simulink model "SparkEV"  (R2022b)
settings: configuration reference "VehicleVariableDae" (kept outside this file)
StartFcn:
  | %tic
StopFcn:
  | %toc
undefined symbols (not defined in the file): CtrlTcuInitGear, CtrlVcuCltch1InitCmd, Disabled, DriverPreviewDist, EnvAbsPrs, EnvAirTemp, EnvGrvty, EnvNomFrictionScaling, EnvNominalGrade, EnvWindVelX, EnvWindVelY, EnvWindVelZ, PlntVehDstCGFrntAxl, PlntVehDstCGRearAxl, PlntVehInitLatPos, PlntVehInitLongPos, PlntVehInitPitchAng, PlntVehInitRollAng, PlntVehInitVertPos, PlntVehInitYawAng, PlntVehMass, PlntVehTrckWdth, PlntVehYawMomentInertia, ScnCRMaxLatAccel, ScnCRRadius, ScnDLCGateLongPos, ScnDLCLatRef, ScnDLCLatRefOffset, ScnDLCLongRefBpt, ScnDLCLongRefStartPos, ScnDLCVehicleWidth, ScnFHCounterDwellTime, ScnFHInitialDwellTime, ScnFHReturnTime, ScnFHRollRateZeroCross, ScnFHSteerAmp, ScnFHSteerSpeed, ScnISHandwheelRate, ScnISMaxHandwheelAng, ScnISMaxLatAccel, ScnISSteerHoldTime, ScnLongVelRef, ScnSDDwellTime, ScnSDSteerAmp, ScnSDSteerFreq, ScnSimTime, ScnSSFinalFreq, ScnSSSteerAmp, ScnSSSweepTime, ScnStartTime, US06
libraries: simulink x13, vehdynlibscenariocommon x7, vehdynlibviscommon x3, autolibshared x2, sim3dgroundtruthsensorlib x2, vehdynlibdriver x1, sharedtransform x1, sim3dlib x1, sim3dautolib x1
(part 3 of 4)

== system SparkEV/Driver Commands/Driver Commands/Open Loop ==
  VehFdbk : Inport
  SteerCmd : Inport  Port=2
  AccelCmd : Inport  Port=3
  BrakeCmd : Inport  Port=4
  GearCmd : Inport  Port=5
  Bus Creator1 : BusCreator  Inputs=5
  Constant : Constant  Value=false
  Signal Specification : SignalSpecification  Unit=1
  Signal Specification1 : SignalSpecification  Unit=1
  Signal Specification2 : SignalSpecification  Unit=1
  Terminator : Terminator
  Unit Conversion : UnitConversion
  Wheel Angle Limit * Steer Ratio : Gain  Gain=40*pi/180*18
  Driver : Outport  VectorParamsAs1DForOutWhenUnconnected=off
  wires:
  Signal Specification2/1 -> Bus Creator1/4  "GearCmd"
  BrakeCmd/1 -> Signal Specification1/1
  Wheel Angle Limit * Steer Ratio/1 -> Bus Creator1/1  "SteerCmd"
  Bus Creator1/1 -> Driver/1
  Unit Conversion/1 -> Wheel Angle Limit * Steer Ratio/1
  AccelCmd/1 -> Signal Specification/1
  VehFdbk/1 -> Terminator/1
  SteerCmd/1 -> Unit Conversion/1
  Signal Specification/1 -> Bus Creator1/2  "AccelCmd"
  GearCmd/1 -> Signal Specification2/1
  Signal Specification1/1 -> Bus Creator1/3  "DecelCmd"
  Constant/1 -> Bus Creator1/5  "IgnSwtch"

== system SparkEV/Driver Commands/Driver Commands/Predictive Driver ==
  VehRef : Inport
  VehFdbk : Inport  Port=2
  Env : Inport  Port=3
  Bus Creator1 : BusCreator  Inputs=5
  Bus Selector : BusSelector  OutputSignals=Body.InertFrm.Cg.Disp.Y,Body.BdyFrm.Cg.Vel.ydot,Body.InertFrm.Cg.Ang.psi,Body.BdyFrm.Cg.AngVel.r
  Bus Selector1 : BusSelector  OutputSignals=LngRef,LtrlRef,EnblSteerCmd,SteerOvrCmd,SteerHld,SteerZero,EnblAccelOvr,AccelOvrCmd,AccelHld,AccelZero,EnblDecelCmd,DecelOvrCmd,DecelHld,DecelZero
  Constant : Constant  Value=false
  Hill Hold : Subsystem
  Linear Predictive Driver : vehdynlibdriver/Predictive Driver  extAccelOvr=on  extDecelOvr=on  extAccelHld=on  extDecelHld=on  extAccelZero=on  extDecelZero=on  extSteerOvr=on  extSteerHld=on  extSteerZero=on  cntrlType=Predictive  cntrlTypeLat=Predictive  shftType=Reverse, Neutral, Drive  coordMode=SAE J670 (Z-down)  refType=Reference pose  velUnits=m/s  angUnits=rad  gearOut=on  steerOut=on  Kp=3  Ki=1  Kff=1  Kg=0  VehVelVec=[0 100]  KffVec=[.1 .1]  KpVec=[10 10]  KiVec=[5 5]  KgVec=[0 0]  vnom=5  Kaw=1  tauerr=.075  tau=DriverTimeConst  L=DriverPreviewDist  Kpt=DriverTractiveForce  aR=DriverRollRes  bR=DriverDrivelineRes  cR=DriverAeroRes  g=EnvGrvty  vecPose=off  dynamMode=off  PositionGainF=2.5  PositionGainR=2.5  YawRateGain=.2  DelayGain=.2  enableDrift=off  BetaRef=10  KpBeta=1  KpDrift=1  KdDrift=1  KpPsi=1  KOmega=.1  tOmega=.1  a=PlntVehDstCGFrntAxl  b=PlntVehDstCGRearAxl  m=PlntVehMass  Cy_f=DriverFrontCornerStiff  Cy_r=DriverRearCornerStiff  I=PlntVehYawMomentInertia  Ksteer=PlntSteerRatio  theta=DriverWheelRange  Idl=1  Re=PlntWhlLdRadius  lambda_mu=1  GearInit=DriverInitialGear  tShift=DriverShiftTime  pdlVec=[0.1 0.4 0.5 0.9]  upShftTbl=[-1 12.9375 26.4375 39.9375 51.18749999999999 62.4375 72.84375 83.25;-1 16.3125 29.8125 43.3125 54.5624 65.8125 76.78125 87.75;-1 19.6875 33.1875 46.68749999999999 57.9375 69.1875 80.71875 92.25;-1 33 52.5 77.25 100.5 138.75 161.875 185]  dwnShftTbl=[-1 12.9375 26.4375 39.9375 51.18749999999999 62.4375 72.84375 83.25;-1 16.3125 29.8125 43.3125 54.5624 65.8125 76.78125 87.75;-1 19.6875 33.1875 46.68749999999999 57.9375 69.1875 80.71875 92.25;-1 33 52.5 77.25 100.5 138.75 161.875 185]  tClutch=.5  tRev=.5  tPark=120  UpGearVec="[0  1  2  3  4  5  6  7]"  DownGearVec="[1  2  3  4  5  6  7  8]"  aMode=2
  Terminator : Terminator
  Unit Conversion : UnitConversion
  Driver : Outport  VectorParamsAs1DForOutWhenUnconnected=off
  wires:
  Linear Predictive Driver/3 -> Bus Creator1/2  "AccelCmd"
  Bus Selector/2 -> Linear Predictive Driver/18  "<ydot>"
  Bus Selector/1 -> Linear Predictive Driver/17  "<Y>"
  Bus Selector1/10 -> Linear Predictive Driver/10  "<AccelZero>"
  Bus Creator1/1 -> Driver/1
  Linear Predictive Driver/1 -> Terminator/1
  Bus Selector/3 -> Linear Predictive Driver/19  "<psi>"
  VehFdbk/1 -> Hill Hold/7(VehFdbk), Bus Selector/1
  Bus Selector1/2 -> Linear Predictive Driver/2  "<LtrlRef>"
  Bus Selector/4 -> Linear Predictive Driver/20  "<r>"
  VehRef/1 -> Bus Selector1/1
  Bus Selector1/1 -> Unit Conversion/1  "<LngRef>"
  Linear Predictive Driver/2 -> Bus Creator1/1  "SteerCmd"
  Linear Predictive Driver/4 -> Bus Creator1/3  "DecelCmd"
  Linear Predictive Driver/5 -> Bus Creator1/4  "GearCmd"
  Constant/1 -> Bus Creator1/5  "IgnSwtch"
  Bus Selector1/3 -> Linear Predictive Driver/3  "<EnblSteerCmd>"
  Bus Selector1/4 -> Linear Predictive Driver/4  "<SteerOvrCmd>"
  Bus Selector1/5 -> Linear Predictive Driver/5  "<SteerHld>"
  Bus Selector1/6 -> Linear Predictive Driver/6  "<SteerZero>"
  Bus Selector1/7 -> Linear Predictive Driver/7  "<EnblAccelOvr>"
  Bus Selector1/8 -> Linear Predictive Driver/8  "<AccelOvrCmd>"
  Bus Selector1/9 -> Linear Predictive Driver/9  "<AccelHld>"
  Bus Selector1/11 -> Hill Hold/2(<EnblDecelCmd>)  "<EnblDecelCmd>"
  Bus Selector1/12 -> Hill Hold/3(<DecelOvrCmd>)  "<DecelOvrCmd>"
  Bus Selector1/13 -> Hill Hold/4(<DecelHld>)  "<DecelHld>"
  Bus Selector1/14 -> Hill Hold/5(<DecelZero>)  "<DecelZero>"
  Env/1 -> Hill Hold/6(Env)
  Hill Hold/5(Grade) -> Linear Predictive Driver/15
  Hill Hold/6(VelFdbk) -> Linear Predictive Driver/16
  Hill Hold/4(DecelZero) -> Linear Predictive Driver/14
  Hill Hold/3(DecelHld) -> Linear Predictive Driver/13
  Hill Hold/2(DecelOvrCmd) -> Linear Predictive Driver/12
  Hill Hold/1(EnblDecelOvr) -> Linear Predictive Driver/11
  Unit Conversion/1 -> Linear Predictive Driver/1, Hill Hold/1(LngRef)

== system SparkEV/Environment/Ground Feedback/3D Engine ==
  Friction : Inport
  WheelFdbk : Inport  Port=2
  3D Engine Source : Subsystem  Variant=on  VariantControl=Choice  mask(Terrain Source){terrType=Single point}
      mask prompts: terrType "Terrain feedback type:"
      mask help:
      | This variant subsystem provides the option for:
      | - a single point of contact for each wheel with minimal post-processing ideal for smooth surfaces and maximum run-time performance.
      | - multiple points of contact per wheel which may be used when interested in non-smooth terrain at a higher computational cost and requires Vehicle Dynamics Blockset.
      mask TypeOptions terrType: Single point | Multiple points
  Bus Creator2 : BusCreator  Inputs=4
  Bus Creator3 : BusCreator  Inputs=3
  Demux1 : Demux
  Signal Specification1 : SignalSpecification  Unit=1
  Ground : Outport  VectorParamsAs1DForOutWhenUnconnected=off
  wires:
  Signal Specification1/1 -> Demux1/1
  Demux1/1 -> Bus Creator2/1  "mu_FL"
  Demux1/3 -> Bus Creator2/3  "mu_RL"
  Demux1/4 -> Bus Creator2/4  "mu_RR"
  Demux1/2 -> Bus Creator2/2  "mu_FR"
  Bus Creator2/1 -> Bus Creator3/3  "mu"
  Bus Creator3/1 -> Ground/1
  Friction/1 -> Signal Specification1/1
  WheelFdbk/1 -> 3D Engine Source/1(WheelFdbk)
  3D Engine Source/1(z) -> Bus Creator3/1  "z"
  3D Engine Source/2(DCM) -> Bus Creator3/2  "DCM"

== system SparkEV/Environment/Ground Feedback/Constant ==
  Friction : Inport
  Bus Creator : BusCreator  Inputs=4
  Bus Creator2 : BusCreator  Inputs=4
  Bus Creator3 : BusCreator  Inputs=3
  Constant1 : Constant  Value=zeros(4,1)
  Constant2 : Constant  Value=repmat(eye(3),1,1,4)  SampleTime=-1
  Demux : Demux
  Demux1 : Demux
  Signal Specification : SignalSpecification  Unit=m
  Signal Specification1 : SignalSpecification  Unit=1
  Ground : Outport  VectorParamsAs1DForOutWhenUnconnected=off
  wires:
  Constant1/1 -> Signal Specification/1
  Signal Specification/1 -> Demux/1
  Demux/4 -> Bus Creator/4  "G_RR_z"
  Demux/1 -> Bus Creator/1  "G_FL_z"
  Demux/3 -> Bus Creator/3  "G_RL_z"
  Demux/2 -> Bus Creator/2  "G_FR_z"
  Bus Creator/1 -> Bus Creator3/1  "z"
  Demux1/3 -> Bus Creator2/3  "mu_RL"
  Demux1/4 -> Bus Creator2/4  "mu_RR"
  Demux1/1 -> Bus Creator2/1  "mu_FL"
  Demux1/2 -> Bus Creator2/2  "mu_FR"
  Bus Creator2/1 -> Bus Creator3/3  "mu"
  Friction/1 -> Signal Specification1/1
  Signal Specification1/1 -> Demux1/1
  Bus Creator3/1 -> Ground/1
  Constant2/1 -> Bus Creator3/2  "DCM"

== system SparkEV/Environment/Varying Friction/Constant Friction ==
  Friction Scaling : Constant  Value=ones(4,1).*EnvNomFrictionScaling  SampleTime=0
  FricCoeffLambda : Outport
  wires:
  Friction Scaling/1 -> FricCoeffLambda/1

== system SparkEV/Environment/Varying Friction/Varying Friction ==
  In1 : Inport
  In2 : Inport  Port=2
  Cg : Inport  Port=3
  Bus Selector : BusSelector  OutputSignals=FrntAxl.Lft.Disp.X,FrntAxl.Rght.Disp.X,RearAxl.Lft.Disp.X,RearAxl.Rght.Disp.X
  Bus Selector1 : BusSelector  OutputSignals=FrntAxl.Lft.Disp.Y,FrntAxl.Rght.Disp.Y,RearAxl.Lft.Disp.Y,RearAxl.Rght.Disp.Y
  Road Track Friction : Subsystem  mask(Road Track Friction){surface_popup=Split friction coefficient scaling factor, lambda_g=EnvNomFrictionScaling, lambda_r=.6, r_x0=175, r_y0=-100, r_xw=1000, r_yw=500, aMode=2}
      mask prompts: surface_popup "Type of surface:"; lambda_g "Scaling factor for the friction coefficient of ground, lambda_g :"; lambda_r "Scaling factor for the friction coefficient of rectangular surface, lambda_r :"; r_x0 "X coordinate of lower left corner of rectangular surface, r_x0 [m]:"; r_y0 "Y coordinate of lower left corner of rectangular surface, r_y0 [m]:"; r_xw "Rectangular surface width in X direction, r_xw [m]:"; r_yw "Rectangular surface width in Y direction, r_yw [m]:"
      mask init:
      | % Scaling factor for the friction coefficient around the rectangular region
      | mutable = [lambda_g, lambda_g, lambda_g, lambda_g;
      |            lambda_g, lambda_r, lambda_r, lambda_g; 
      |            lambda_g, lambda_r, lambda_r, lambda_g; 
      |            lambda_g, lambda_g, lambda_g, lambda_g ];
      |        
      | 
      | % The step is distance between breakpoint near the boundary of high and
      | % low friction coefficient
      | 
      | step = 0.01 ; 
      | 
      | % In the mask initialization, xbr and ybr breakpoints are with respect to
      | % Body fixed coordinate system. At time t=0, xbr and ybr breakpoints
      | % updates to Earth (Inertial) Fixed coordinate system. The breakpoints for
      | % the lookup table are added via inputs.
      | 
      | xbr = [(r_x0 - step) , (r_x0 + step), (r_x0 + r_xw - step) , (r_x0 + r_xw + step) ];
      | ybr = [(r_y0 - step) , (r_y0 + step), (r_y0 + r_yw - step) , (r_y0 + r_yw + step) ];
      | 
      | 
      | % To check if the created track is split mu or constant mu
      | 
      | surface_popup = get_param(gcb, 'surface_popup');
      | 
      | if strcmp(surface_popup, 'Split friction coefficient scaling factor')
      |     SplitLambdaTrck = 1;
      | elseif strcmp(surface_popup, 'Constant friction coefficient scaling factor')
      |     SplitLambdaTrck = 0;
      | end
      mask Help: eval('vdynblkshelp(''vdynblkstrack'')');
      mask TypeOptions surface_popup: Constant friction coefficient scaling factor | Split friction coefficient scaling factor
      mask Callback surface_popup:
      | surface_popup = get_param(gcb, 'surface_popup');
      | m = Simulink.Mask.get(gcb);
      | 
      | lambda_g = m.getParameter('lambda_g');
      | lambda_r = m.getParameter('lambda_r');
      | r_x0 = m.getParameter('r_x0');
      | r_y0 = m.getParameter('r_y0');
      | r_xw = m.getParameter('r_xw');
      | r_yw = m.getParameter('r_yw');
      | %track_view = m.getParameter('track_view');
      | 
      | 
      | if strcmp(surface_popup, 'Split friction coefficient scaling factor')
      |     lambda_g.Visible = 'on';
      |     lambda_r.Visible = 'on';
      |     r_x0.Visible = 'on';
      |     r_y0.Visible = 'on';
      |     r_xw.Visible = 'on';
      |     r_yw.Visible = 'on';
      |     %track_view.Visible = 'on';
      | 
      | elseif strcmp(surface_popup,'Constant friction coefficient scaling factor')
      |     lambda_g.Visible = 'on';
      |     lambda_r.Visible = 'off';
      |     r_x0.Visible = 'off';
      |     r_y0.Visible = 'off';
      |     r_xw.Visible = 'off';
      |     r_yw.Visible = 'off';
      |     %track_view.Visible = 'off';
      | end
      | [~]=autosharedicon('autolibutils',gcb,0);
      mask DialogControl DescGroupVar Prompt: Track description  (mask)
      mask DialogControl DescTextVar Prompt: Generates a default or user-specified track which creates a rectangular surface of specified friction coefficient. The location of rectangular surface is relative to the origin of Body Fixed Coordinate System.The input of the block is X and Y coordinates of the wheel from the vehicle feedback bus. The block output is friction coefficient for all the wheels.
  Wheel Coordinates : Subsystem
  FricCoeffLambda : Outport
  wires:
  Bus Selector1/1 -> Wheel Coordinates/5(FrntAxlLftY)  "<Y>"
  Bus Selector/3 -> Wheel Coordinates/3(RearAxlLftX)  "<X>"
  Bus Selector/4 -> Wheel Coordinates/4(RearAxlRghtX)  "<X>"
  Wheel Coordinates/1(XWhl) -> Road Track Friction/1(XWhl)
  Bus Selector1/2 -> Wheel Coordinates/6(FrntAxlRghtY)  "<Y>"
  Bus Selector/2 -> Wheel Coordinates/2(FrntAxlRghtX)  "<X>"
  Bus Selector/1 -> Wheel Coordinates/1(FrntAxlLftX)  "<X>"
  Bus Selector1/3 -> Wheel Coordinates/7(RearAxlLftY)  "<Y>"
  Bus Selector1/4 -> Wheel Coordinates/8(RearAxlRghtY)  "<Y>"
  Cg/1 -> Road Track Friction/3(Cg)
  Wheel Coordinates/2(YWhl) -> Road Track Friction/2(YWhl)
  Road Track Friction/1(FricCoeffLambda) -> FricCoeffLambda/1
  In1/1 -> Bus Selector/1
  In2/1 -> Bus Selector1/1

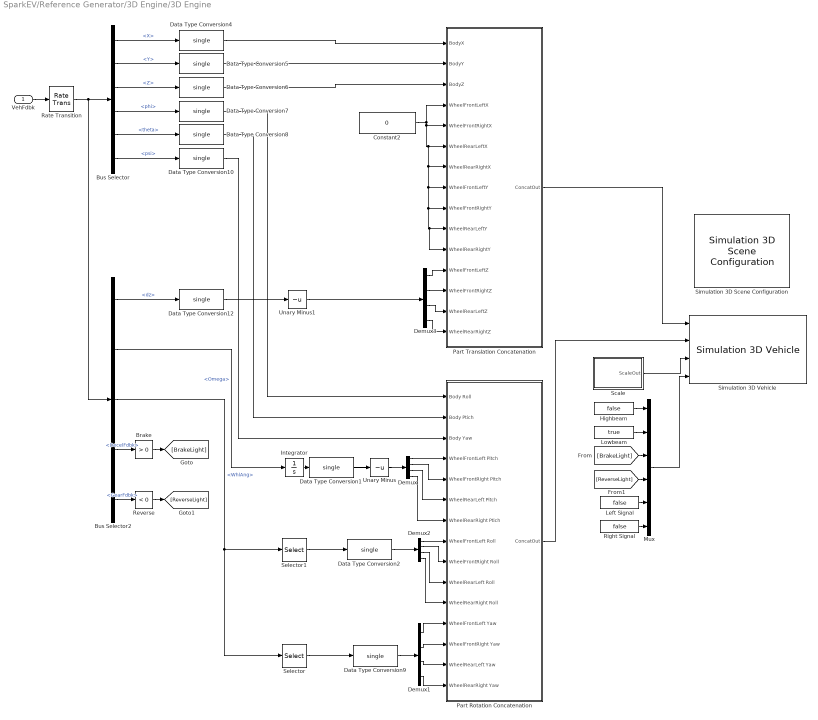
== system SparkEV/Reference Generator/3D Engine/3D Engine ==
  VehFdbk : Inport
  Brake : simulink/Logic and Bit Operations/Compare To Constant  relop=>  const=0  OutDataTypeStr=boolean  ZeroCross=off
  Bus Selector : BusSelector  OutputSignals=Body.InertFrm.Geom.Disp.X,Body.InertFrm.Geom.Disp.Y,Body.InertFrm.Geom.Disp.Z,Body.InertFrm.Cg.Ang.phi,Body.InertFrm.Cg.Ang.theta,Body.InertFrm.Cg.Ang.psi
  Bus Selector2 : BusSelector  OutputSignals=Suspension.SuspWheel.dz,Wheels.Wheels.Omega,Suspension.SuspWheel.WhlAng,Driver.DecelFdbk,Driver.GearFdbk
  Constant2 : Constant  Value=0  OutDataTypeStr=single
  Data Type Conversion{1..2,4..10,12} (10 alike) : DataTypeConversion  OutDataTypeStr=single  SaturateOnIntegerOverflow=off  RndMeth=Floor
  Demux{,1..3} (4 alike) : Demux
  Highbeam : Constant  Value=false
  Integrator : Integrator  WrapState=on  WrappedStateUpperValue=2*pi  WrappedStateLowerValue=0  ZeroCross=off
  Left Signal : Constant  Value=false
  Lowbeam : Constant  Value=true
  Mux : Mux  Inputs=6
  Part Rotation Concatenation : Subsystem
  Part Translation Concatenation : Subsystem
  Rate Transition : RateTransition  OutPortSampleTime=dt3D
  Reverse : simulink/Logic and Bit Operations/Compare To Constant  relop=<  const=0  OutDataTypeStr=boolean  ZeroCross=off
  Right Signal : Constant  Value=false
  Scale : Subsystem
  Selector : Selector  NumberOfDimensions=2  InputPortWidth=3  IndexOptions=Index vector (dialog),Select all  Indices=[3],1  OutputSizes=1,1
  Selector1 : Selector  NumberOfDimensions=2  InputPortWidth=3  IndexOptions=Index vector (dialog),Select all  Indices=[1],1  OutputSizes=1,1
  Simulation 3D Scene Configuration : sim3dlib/Simulation 3D Scene Configuration  Priority=0  ProjectFormat=Default Scenes  SceneDesc=Open surface  ProjectName=C:\Program Files\MATLAB\R2022b\toolbox\shared\sim3d_projects\automotive_project\UE4\WindowsNoEditor\VehicleSimulation.exe  ScenePath=/Game/Maps/HwStrght  EnableOpenDRIVE=off  vehTagList={'Scene Origin'}  vehTag=Scene Origin  OpVisEn=off  Ts=dt3D  EnableWindow=on  EnableRemoteAccess=off  EnableWeather=off  SunAltitude=40.0  SunAzimuth=90  clouds=10  wind=1  fog=0  rain=0  EnableGeospatial=off  OriginHeight=200  OriginLatitude=40.744652  OriginLongitude=-73.988864  MapStyle=Aerial  AdditionalAssetIDs=[]  UseAdvancedSunSky=off  SolarTime=11  TimeZone=-5  Day=21  Month=9  Year=2022  UseDaylightSavingTime=on  DSTStartDay=10  DSTStartMonth=3  DSTEndDay=3  DSTEndMonth=11  DSTSwitchHour=2  sensorTag=MainCamera1  sensorId=1  sensorName=MainCamera1  mountLoc=Origin  offsetFlag=off  tmountOffset=[0, 0, 0]  rmountOffset=[0, 0, 0]  HorizontalResolution=1280  VerticalResolution=720  HorizontalFOV=60  mountPoint=[0 0 0]  mountOrientation=[0 0 0]  aMode=2  ID=1  GeoTrigger=Inactive
      settings: LibrarySourceBlock=vdynlib/Vehicle Scenarios/Sim3D/Sim3D Core/Simulation 3D Scene Configuration
  Simulation 3D Vehicle : sim3dautolib/Simulation 3D Vehicle  Priority=-1  PassVehMesh=Muscle car  MeshPath=/MathWorksSimulation/Vehicles/Muscle/Meshes/SK_MuscleCar.SK_MuscleCar  VehColor=Red  ActorName=SimulinkVehicle1  VehLightsControl=on  HeadlightColor=[ 1, 1, 1 ]  HighBeamIntensity=100000  LowBeamIntensity=60000  HighBeamConeAngle=1.22  LowBeamConeAngle=1.22  LeftHeadlightOrientation=[ 0, 0 ]  RightHeadlightOrientation=[ 0, 0 ]  BrakelightIntensity=500  ReverselightIntensity=500  SignallightIntensity=500  SignallightPeriod=1  SignalPulseWidth=50  Translation=[PlntVehInitLongPos PlntVehInitLatPos -PlntVehInitVertPos; 0 0 0; 0 0 0; 0 0 0; 0 0 0]  Rotation=[PlntVehInitRollAng PlntVehInitPitchAng PlntVehInitYawAng; 0 0 0; 0 0 0; 0 0 0; 0 0 0]  Scale=ones( 5, 3 )  SampleTime=dt3D  ActorType=SimulinkVehicle  ID=1  aMode=2  ActorTag=SimulinkVehicle1
  Unary Minus : UnaryMinus
  Unary Minus1 : UnaryMinus
  wires:
  Unary Minus/1 -> Demux/1
  Unary Minus1/1 -> Demux3/1
  Selector1/1 -> Data Type Conversion2/1
  Selector/1 -> Data Type Conversion9/1
  Bus Selector2/5 -> Reverse/1  "<GearFdbk>"
  Bus Selector2/4 -> Brake/1  "<DecelFdbk>"
  Left Signal/1 -> Mux/5
  Right Signal/1 -> Mux/6
  Lowbeam/1 -> Mux/2
  [ReverseLight] -> Mux/4
  Reverse/1 -> [ReverseLight]
  Highbeam/1 -> Mux/1
  Brake/1 -> [BrakeLight]
  Mux/1 -> Simulation 3D Vehicle/4
  [BrakeLight] -> Mux/3
  Bus Selector/3 -> Data Type Conversion6/1  "<Z>"
  Bus Selector/5 -> Data Type Conversion8/1  "<theta>"
  Bus Selector/6 -> Data Type Conversion10/1  "<psi>"
  Bus Selector/2 -> Data Type Conversion5/1  "<Y>"
  Bus Selector/1 -> Data Type Conversion4/1  "<X>"
  Data Type Conversion7/1 -> Part Rotation Concatenation/1(Body Roll)
  Data Type Conversion4/1 -> Part Translation Concatenation/1(BodyX)
  Constant2/1 -> Part Translation Concatenation/4(WheelFrontLeftX), Part Translation Concatenation/11(WheelRearRightY), Part Translation Concatenation/10(WheelRearLeftY), Part Translation Concatenation/9(WheelFrontRightY), Part Translation Concatenation/8(WheelFrontLeftY), Part Translation Concatenation/7(WheelRearRightX), Part Translation Concatenation/6(WheelRearLeftX), Part Translation Concatenation/5(WheelFrontRightX)
  Data Type Conversion10/1 -> Part Rotation Concatenation/3(Body Yaw)
  Data Type Conversion5/1 -> Part Translation Concatenation/2(BodyY)
  Data Type Conversion8/1 -> Part Rotation Concatenation/2(Body Ptich)
  Data Type Conversion1/1 -> Unary Minus/1
  Integrator/1 -> Data Type Conversion1/1
  Demux1/2 -> Part Rotation Concatenation/13(WheelFrontRight Yaw)
  Demux1/1 -> Part Rotation Concatenation/12(WheelFrontLeft Yaw)
  Data Type Conversion9/1 -> Demux1/1
  Bus Selector2/2 -> Integrator/1  "<Omega>"
  Bus Selector2/3 -> Selector/1, Selector1/1  "<WhlAng>"
  Demux2/4 -> Part Rotation Concatenation/11(WheelRearRight Roll)
  Demux2/3 -> Part Rotation Concatenation/10(WheelRearLeft Roll)
  Demux2/2 -> Part Rotation Concatenation/9(WheelFrontRight Roll)
  Demux2/1 -> Part Rotation Concatenation/8(WheelFrontLeft Roll)
  Demux1/3 -> Part Rotation Concatenation/14(WheelRearLeft Yaw)
  Demux1/4 -> Part Rotation Concatenation/15(WheelRearRight Yaw)
  Data Type Conversion6/1 -> Part Translation Concatenation/3(BodyZ)
  VehFdbk/1 -> Rate Transition/1
  Demux3/2 -> Part Translation Concatenation/13(WheelFrontRightZ)
  Demux3/1 -> Part Translation Concatenation/12(WheelFrontLeftZ)
  Demux3/3 -> Part Translation Concatenation/14(WheelRearLeftZ)
  Demux3/4 -> Part Translation Concatenation/15(WheelRearRightZ)
  Data Type Conversion12/1 -> Unary Minus1/1
  Part Translation Concatenation/1(ConcatOut) -> Simulation 3D Vehicle/1
  Part Rotation Concatenation/1(ConcatOut) -> Simulation 3D Vehicle/2
  Bus Selector/4 -> Data Type Conversion7/1  "<phi>"
  Data Type Conversion2/1 -> Demux2/1
  Demux/1 -> Part Rotation Concatenation/4(WheelFrontLeft Pitch)
  Demux/2 -> Part Rotation Concatenation/5(WheelFrontRight Pitch)
  Demux/3 -> Part Rotation Concatenation/6(WheelRearLeft Pitch)
  Demux/4 -> Part Rotation Concatenation/7(WheelRearRight Ptich)
  Scale/1(ScaleOut) -> Simulation 3D Vehicle/3
  Rate Transition/1 -> Bus Selector2/1, Bus Selector/1
  Bus Selector2/1 -> Data Type Conversion12/1  "<dz>"

== system SparkEV/Reference Generator/3D Engine/3D Engine Disabled ==
  VehFdbk : Inport
  Terminator : Terminator
  wires:
  VehFdbk/1 -> Terminator/1

== system SparkEV/Reference Generator/Reference Generator/Braking ==
  "VehFdbk " : Inport
  Bus Creator : BusCreator  Inputs=3
  Bus Creator1 : BusCreator  Inputs=14
  Constant{,2..3,8} (4 alike) : Constant  Value=0
  Constant{1,4..7,9..12} (9 alike) : Constant  Value=false
  Ground : Ground
  Ground1 : Ground
  Ground2 : Ground
  Signal Specification : SignalSpecification  Unit=rad
  Signal Specification1 : SignalSpecification  Unit=one
  Signal Specification2 : SignalSpecification  Unit=one
  Straight Maneuver Reference Generator : vehdynlibscenariocommon/Straight Maneuver Reference Generator  t_start=.5  ax=0.5  xdot_r=20  xdotUnit=mph  brakingParam=Longitudinal displacement  t_brake=15  x_brake=200  ax_dec=1  BufferSize=40960  fixhw=on  faultTracking=on  xdot_rmax=1  xdot_rmean=2  r_max=1  hw_max=3  SimStopOnFault=off  aMode=2
  " Vis" : Outport
  " Ref" : Outport  Port=2
  " Fdbk" : Outport  Port=3
  wires:
  Straight Maneuver Reference Generator/1 -> Bus Creator1/1  "XRef"
  Ground/1 -> Bus Creator/1  "XRef"
  Ground2/1 -> Bus Creator/3  "ZRef"
  Constant6/1 -> Bus Creator1/7  "EnblAccelOvr"
  Constant/1 -> Bus Creator1/2  "LtrlRef"
  Bus Creator1/1 -> " Ref"/1
  Constant5/1 -> Bus Creator1/6  "SteerZero"
  Constant3/1 -> Signal Specification/1
  Constant7/1 -> Bus Creator1/9  "AccelHld"
  Signal Specification1/1 -> Bus Creator1/8  "AccelOvrCmd"
  Ground1/1 -> Bus Creator/2  "YRef"
  Signal Specification/1 -> Bus Creator1/4  "SteerOvrCmd"
  Bus Creator/1 -> " Vis"/1
  Constant12/1 -> Bus Creator1/14  "DecelZero"
  Constant1/1 -> Bus Creator1/3  "EnblSteerCmd"
  Constant10/1 -> Bus Creator1/11  "EnblDecelCmd"
  Constant11/1 -> Bus Creator1/13  "DecelHld"
  Signal Specification2/1 -> Bus Creator1/12  "DecelOvrCmd"
  Constant2/1 -> Signal Specification2/1
  Constant8/1 -> Signal Specification1/1
  Constant4/1 -> Bus Creator1/5  "SteerHld"
  Constant9/1 -> Bus Creator1/10  "AccelZero"
  "VehFdbk "/1 -> Straight Maneuver Reference Generator/1, " Fdbk"/1

== system SparkEV/Reference Generator/Reference Generator/Double Lane Change ==
  "VehFdbk " : Inport
  Double Lane Change : vehdynlibscenariocommon/Lane Change Reference Generator  VariantControl=Variant1  ssMode=Initialize from model  ssVar=dlcSS35mph  t_start=t_start  XGate=XGate  xdot_r=xdot_r  xdotUnit=mph  xStart=xStart  vehW=vehW  latoff=latoff  lattoff=VEH.InitialLatPosition  centerSwitch=on  xSimStop=off  ssDefault=off  latRefbp=latRefbp  latRef=latRef  X_o=X_o  Y_o=Y_o  psi_o=phi_o  ssTol=1e-3  ssMaxTime=30  ssWSName=dlcSS35mph  aMode=2  use3DCones=off
      link override ISO 3888-2/Lateral Reference: LabelModeActiveChoice=1
  " Vis" : Outport  VectorParamsAs1DForOutWhenUnconnected=off
  " Ref" : Outport  Port=2  VectorParamsAs1DForOutWhenUnconnected=off
  " Fdbk" : Outport  Port=3  VectorParamsAs1DForOutWhenUnconnected=off
  wires:
  "VehFdbk "/1 -> " Fdbk"/1, Double Lane Change/1
  Double Lane Change/1 -> " Vis"/1
  Double Lane Change/2 -> " Ref"/1

== system SparkEV/Reference Generator/Reference Generator/Drive Cycle ==
  "VehFdbk " : Inport
  Bus Creator : BusCreator  Inputs=3
  Bus Creator1 : BusCreator  Inputs=14
  Constant{,2..3,8,13..15} (7 alike) : Constant  Value=0
  Constant{1,4..7,9..12} (9 alike) : Constant  Value=false
  Drive Cycle Source : autolibshared/Drive Cycle Source  cycleVar=US06  fileVar=L:\Bauto\matlab\test\toolbox\shared\autoblks\scenario\adac.txt  tfinal="600  seconds, Cyclic"  cycleRepeat=on  outAccPort=off  outGearPort=off  gearList=No gear data  t_wot1=1  xdot_woto=0  xdot_wot1=7000  t_wot2=500  xdot_wot2=0  t_wotend=505  srcUnit=m/s  outUnit=mph  srcAccUnit=m/s/s  outAccUnit=m/s^2  dt=0  aMode=6  faultOption=off  velBnd=2  velBndUnit=mph  inUnit=m/s  timeBnd=1  failOption=off  stopSim=off  maxFaultCnt=10  maxFaultTime=2  maxTotFaultTime=15  traceOption=off  dtTrace=1  traceWindow=10  lastDCname=US06  lastOutUnit=mph  lastDT=0  lastTB=1  lastSB=2  forceCalcBound=off
  Signal Specification : SignalSpecification  Unit=rad
  Signal Specification1 : SignalSpecification  Unit=one
  Signal Specification2 : SignalSpecification  Unit=one
  " Vis" : Outport  VectorParamsAs1DForOutWhenUnconnected=off
  " Ref" : Outport  Port=2  VectorParamsAs1DForOutWhenUnconnected=off
  " Fdbk" : Outport  Port=3  VectorParamsAs1DForOutWhenUnconnected=off
  wires:
  Constant2/1 -> Signal Specification2/1
  Constant8/1 -> Signal Specification1/1
  Constant4/1 -> Bus Creator1/5  "SteerHld"
  Signal Specification2/1 -> Bus Creator1/12  "DecelOvrCmd"
  Constant12/1 -> Bus Creator1/14  "DecelZero"
  Constant6/1 -> Bus Creator1/7  "EnblAccelOvr"
  Constant7/1 -> Bus Creator1/9  "AccelHld"
  Constant9/1 -> Bus Creator1/10  "AccelZero"
  Signal Specification1/1 -> Bus Creator1/8  "AccelOvrCmd"
  Constant11/1 -> Bus Creator1/13  "DecelHld"
  Constant10/1 -> Bus Creator1/11  "EnblDecelCmd"
  Constant5/1 -> Bus Creator1/6  "SteerZero"
  Signal Specification/1 -> Bus Creator1/4  "SteerOvrCmd"
  Constant3/1 -> Signal Specification/1
  Constant1/1 -> Bus Creator1/3  "EnblSteerCmd"
  Constant/1 -> Bus Creator1/2  "LtrlRef"
  Drive Cycle Source/1 -> Bus Creator1/1  "LngRef"
  Bus Creator1/1 -> " Ref"/1
  "VehFdbk "/1 -> " Fdbk"/1
  Bus Creator/1 -> " Vis"/1
  Constant15/1 -> Bus Creator/3  "ZRef"
  Constant14/1 -> Bus Creator/2  "YRef"
  Constant13/1 -> Bus Creator/1  "XRef"

== system SparkEV/Reference Generator/Reference Generator/Fishhook ==
  "VehFdbk " : Inport
  Bus Creator : BusCreator  Inputs=3
  Constant : Constant  Value=0
  Constant1 : Constant  Value=0
  Constant2 : Constant  Value=0
  Fishhook : vehdynlibscenariocommon/Fishhook  ssMode=Initialize from model  ssVar=fh50mph  t_start=t_start  xdot_r=xdot_r  xdotUnit=mph  steerRate=steerRate  steerA=steerAFH  pFdbk=off  tDwell1=tDwell1  tDwell2=tDwell2  tSteer3=tSteer3  pZero=pZero  steerDir=off  ssDefault=off  X_o=0  Y_o=0  psi_o=0  ssTol=1  ssMaxTime=30  ssWSName=fh50mph  aMode=2
  " Vis" : Outport  VectorParamsAs1DForOutWhenUnconnected=off
  " Ref" : Outport  Port=2  VectorParamsAs1DForOutWhenUnconnected=off
  " Fdbk" : Outport  Port=3  VectorParamsAs1DForOutWhenUnconnected=off
  wires:
  Constant/1 -> Bus Creator/1  "XRef"
  Constant1/1 -> Bus Creator/2  "YRef"
  Constant2/1 -> Bus Creator/3  "ZRef"
  Bus Creator/1 -> " Vis"/1
  Fishhook/1 -> " Ref"/1
  "VehFdbk "/1 -> " Fdbk"/1, Fishhook/1

== system SparkEV/Reference Generator/Reference Generator/Increasing Steer ==
  "VehFdbk " : Inport
  Bus Creator : BusCreator  Inputs=3
  Constant : Constant  Value=0
  Constant1 : Constant  Value=0
  Constant2 : Constant  Value=0
  Increasing Steer : vehdynlibscenariocommon/Slowly Increasing Steer  VariantControl=1  ssMode=Initialize from model  ssVar=is50mph  t_start=t_start  xdot_r=xdot_r  xdotUnit=mph  omega_hw=omega_hw  theta_max=theta_max  t_stop=t_stop  ay_max=ay_max  steerDir=off  ay_stop=on  ssDefault=off  X_o=0  Y_o=0  psi_o=0  ssTol=1  ssMaxTime=30  ssWSName=is50mph  aMode=2
  " Vis" : Outport  VectorParamsAs1DForOutWhenUnconnected=off
  " Ref" : Outport  Port=2  VectorParamsAs1DForOutWhenUnconnected=off
  " Fdbk" : Outport  Port=3  VectorParamsAs1DForOutWhenUnconnected=off
  wires:
  "VehFdbk "/1 -> " Fdbk"/1, Increasing Steer/1
  Bus Creator/1 -> " Vis"/1
  Increasing Steer/1 -> " Ref"/1  "LtrlRef"
  Constant2/1 -> Bus Creator/3  "ZRef"
  Constant1/1 -> Bus Creator/2  "YRef"
  Constant/1 -> Bus Creator/1  "XRef"

== system SparkEV/Reference Generator/Reference Generator/Sine with Dwell ==
  "VehFdbk " : Inport
  Bus Creator : BusCreator  Inputs=3
  Constant : Constant  Value=0
  Constant1 : Constant  Value=0
  Constant2 : Constant  Value=0
  Sine With Dwell : vehdynlibscenariocommon/Sine With Dwell  VariantControl=3  ssMode=Initialize from model  ssVar=swd50mph  t_start=t_start  xdot_r=xdot_r  xdotUnit=mph  steerF=steerF  steerA=steerA  tdwell=tdwell  steerDir=off  ssDefault=off  X_o=0  Y_o=0  psi_o=0  ssTol=1  ssMaxTime=30  ssWSName=swd50mph  aMode=2
  " Vis" : Outport  VectorParamsAs1DForOutWhenUnconnected=off
  " Ref" : Outport  Port=2  VectorParamsAs1DForOutWhenUnconnected=off
  " Fdbk" : Outport  Port=3  VectorParamsAs1DForOutWhenUnconnected=off
  wires:
  Sine With Dwell/1 -> " Ref"/1
  "VehFdbk "/1 -> " Fdbk"/1, Sine With Dwell/1
  Bus Creator/1 -> " Vis"/1
  Constant2/1 -> Bus Creator/3  "ZRef"
  Constant1/1 -> Bus Creator/2  "YRef"
  Constant/1 -> Bus Creator/1  "XRef"

== system SparkEV/Reference Generator/Reference Generator/Swept Sine ==
  "VehFdbk " : Inport
  Bus Creator : BusCreator  Inputs=3
  Constant : Constant  Value=0
  Constant1 : Constant  Value=0
  Constant2 : Constant  Value=0
  Swept Sine : vehdynlibscenariocommon/Swept Sine Reference Generator  VariantControl=2  ssMode=Initialize from model  ssVar=ss30mph  t_start=t_start  xdot_r=xdot_r  xdotUnit=mph  theta_hw=theta_hw  theta_hw_final=theta_hw_final  t_sweep=t_sweep  ssDefault=off  X_o=0  Y_o=0  psi_o=0  ssTol=1  ssMaxTime=30  ssWSName=ss30mph  aMode=2
  " Vis" : Outport  VectorParamsAs1DForOutWhenUnconnected=off
  " Ref" : Outport  Port=2  VectorParamsAs1DForOutWhenUnconnected=off
  " Fdbk" : Outport  Port=3  VectorParamsAs1DForOutWhenUnconnected=off
  wires:
  "VehFdbk "/1 -> " Fdbk"/1, Swept Sine/1
  Swept Sine/1 -> " Ref"/1
  Bus Creator/1 -> " Vis"/1
  Constant2/1 -> Bus Creator/3  "ZRef"
  Constant1/1 -> Bus Creator/2  "YRef"
  Constant/1 -> Bus Creator/1  "XRef"

== system SparkEV/Vehicle/Trailer Input/Ground Info Trailer ==
  Env : Inport
  Ground Info 2 AxleTrailer : Subsystem  VariantControl=0
  Ground Info 3 AxleTrailer : Subsystem  VariantControl=1
  Ground : Outport
  Friction : Outport  Port=2

== system SparkEV/Visualization/ISO 15037-1:2006/Disabled ==
  VehFdbk : Inport
  Terminator1 : Terminator
  wires:
  VehFdbk/1 -> Terminator1/1

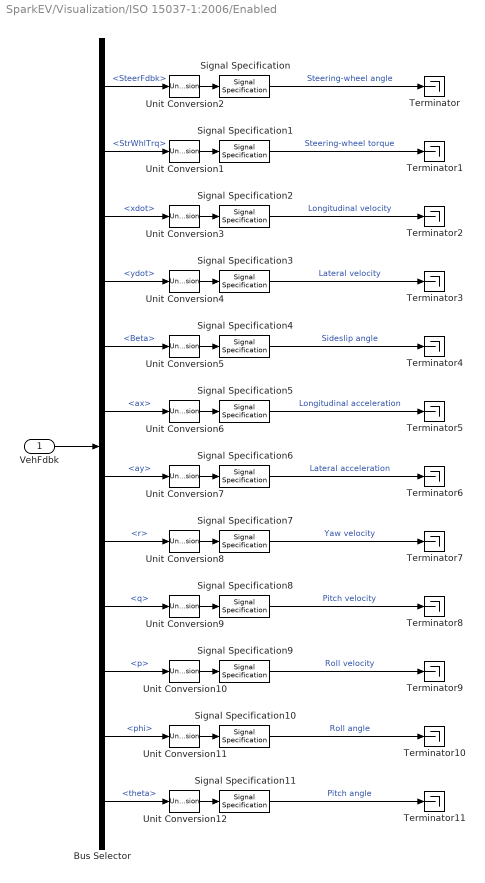
== system SparkEV/Visualization/ISO 15037-1:2006/Enabled ==
  VehFdbk : Inport
  Bus Selector : BusSelector  OutputSignals=Driver.SteerFdbk,Steering.StrWhlTrq,Body.BdyFrm.Cg.Vel.xdot,Body.BdyFrm.Cg.Vel.ydot,Body.BdyFrm.Cg.Ang.Beta,Body.BdyFrm.Cg.Acc.ax,Body.BdyFrm.Cg.Acc.ay,Body.BdyFrm.Cg.AngVel.r,Body.BdyFrm.Cg.AngVel.q,Body.BdyFrm.Cg.AngVel.p,Body.InertFrm.Cg.Ang.phi,Body.InertFrm.Cg.Ang.theta
  Signal Specification{,4,10..11} (4 alike) : SignalSpecification  Unit=deg
  Signal Specification1 : SignalSpecification  Unit=N*m
  Signal Specification2 : SignalSpecification  Unit=km/h
  Signal Specification3 : SignalSpecification  Unit=m/s
  Signal Specification5 : SignalSpecification  Unit=m/s^2
  Signal Specification6 : SignalSpecification  Unit=m/s^2
  Signal Specification7 : SignalSpecification  Unit=deg/s
  Signal Specification8 : SignalSpecification  Unit=deg/s
  Signal Specification9 : SignalSpecification  Unit=deg/s
  Terminator{,1..11} (12 alike) : Terminator
  Unit Conversion{1..12} (12 alike) : UnitConversion
  wires:
  Bus Selector/12 -> Unit Conversion12/1  "<theta>"
  Signal Specification11/1 -> Terminator11/1  "Pitch angle"
  Unit Conversion12/1 -> Signal Specification11/1
  Bus Selector/11 -> Unit Conversion11/1  "<phi>"
  Unit Conversion11/1 -> Signal Specification10/1
  Signal Specification10/1 -> Terminator10/1  "Roll angle"
  Bus Selector/10 -> Unit Conversion10/1  "<p>"
  Signal Specification9/1 -> Terminator9/1  "Roll velocity"
  Unit Conversion10/1 -> Signal Specification9/1
  Bus Selector/9 -> Unit Conversion9/1  "<q>"
  Unit Conversion9/1 -> Signal Specification8/1
  Signal Specification8/1 -> Terminator8/1  "Pitch velocity"
  Bus Selector/8 -> Unit Conversion8/1  "<r>"
  Signal Specification7/1 -> Terminator7/1  "Yaw velocity"
  Unit Conversion8/1 -> Signal Specification7/1
  Bus Selector/7 -> Unit Conversion7/1  "<ay>"
  Unit Conversion7/1 -> Signal Specification6/1
  Signal Specification6/1 -> Terminator6/1  "Lateral acceleration"
  Bus Selector/6 -> Unit Conversion6/1  "<ax>"
  Signal Specification5/1 -> Terminator5/1  "Longitudinal acceleration"
  Unit Conversion6/1 -> Signal Specification5/1
  Bus Selector/5 -> Unit Conversion5/1  "<Beta>"
  Unit Conversion5/1 -> Signal Specification4/1
  Signal Specification4/1 -> Terminator4/1  "Sideslip angle"
  Bus Selector/4 -> Unit Conversion4/1  "<ydot>"
  Signal Specification3/1 -> Terminator3/1  "Lateral velocity"
  Unit Conversion4/1 -> Signal Specification3/1
  Bus Selector/3 -> Unit Conversion3/1  "<xdot>"
  Unit Conversion3/1 -> Signal Specification2/1
  Signal Specification2/1 -> Terminator2/1  "Longitudinal velocity"
  Signal Specification1/1 -> Terminator1/1  "Steering-wheel torque"
  Unit Conversion1/1 -> Signal Specification1/1
  Bus Selector/2 -> Unit Conversion1/1  "<StrWhlTrq>"
  Signal Specification/1 -> Terminator/1  "Steering-wheel angle"
  Unit Conversion2/1 -> Signal Specification/1
  VehFdbk/1 -> Bus Selector/1
  Bus Selector/1 -> Unit Conversion2/1  "<SteerFdbk>"

== system SparkEV/Visualization/Scope Type/DLC ==
  VehFdbk : Inport
  Vis : Inport  Port=2
  Bus Creator : BusCreator  Inputs=3
  Bus Selector3 : BusSelector  OutputSignals=Body.InertFrm.Cg.Disp.X,Body.InertFrm.Cg.Disp.Z
  Bus Selector4 : BusSelector  OutputSignals=LeftBnd,RightBnd,LtrlRef
  Lane Change : Scope
  Mux1 : Mux  Inputs=3
  Rate Transition : RateTransition  OutPortSampleTime=.1
  Rate Transition3 : RateTransition  OutPortSampleTime=.1
  Signal Copy : SignalConversion  OverrideOpt=off
  Signal Copy1 : SignalConversion  OverrideOpt=off
  Signal Copy2 : SignalConversion  OverrideOpt=off
  Ref : Outport  VectorParamsAs1DForOutWhenUnconnected=off
  wires:
  VehFdbk/1 -> Bus Selector3/1
  Vis/1 -> Bus Selector4/1
  Bus Creator/1 -> Ref/1
  Bus Selector3/2 -> Signal Copy2/1  "<Z>"
  Signal Copy/1 -> Bus Creator/2  "YRef"
  Signal Copy1/1 -> Bus Creator/1  "XRef"
  Signal Copy2/1 -> Bus Creator/3  "ZRef"
  Rate Transition3/1 -> Mux1/2  "Right Boundary"
  Bus Selector4/3 -> Signal Copy/1, Mux1/3  "<LtrlRef>"
  Mux1/1 -> Lane Change/1
  Bus Selector4/1 -> Rate Transition/1  "<LeftBnd>"
  Rate Transition/1 -> Mux1/1  "Left Boundary"
  Bus Selector4/2 -> Rate Transition3/1  "<RightBnd>"
  Bus Selector3/1 -> Signal Copy1/1  "<X>"

== system SparkEV/Visualization/Scope Type/None ==
  VehFdbk : Inport
  Vis : Inport  Port=2
  Bus Selector2 : BusSelector  OutputSignals=Driver.SteerFdbk
  Bus Selector9 : BusSelector  OutputSignals=Body.BdyFrm.Cg.AngVel.r
  Signal Specification1 : SignalSpecification  Unit=rad/s
  Signal Specification3 : SignalSpecification  Unit=deg/s
  Unit Conversion4 : UnitConversion
  Yaw Rate and Steer : Scope  NumInputPorts=2
  Ref : Outport  VectorParamsAs1DForOutWhenUnconnected=off
  wires:
  Bus Selector9/1 -> Signal Specification1/1  "<r>"
  Signal Specification3/1 -> Yaw Rate and Steer/1
  Unit Conversion4/1 -> Signal Specification3/1
  VehFdbk/1 -> Bus Selector2/1, Bus Selector9/1  "VehFdbk"
  Bus Selector2/1 -> Yaw Rate and Steer/2  "<SteerFdbk>"
  Vis/1 -> Ref/1
  Signal Specification1/1 -> Unit Conversion4/1

== system SparkEV/Visualization/Scope Type/XYZ ==
  VehFdbk : Inport
  Vis : Inport  Port=2
  Terminator : Terminator
  Ref : Outport  VectorParamsAs1DForOutWhenUnconnected=off
  wires:
  Vis/1 -> Ref/1
  VehFdbk/1 -> Terminator/1

== system SparkEV/Visualization/Vehicle XY Plotter/Disabled ==

== system SparkEV/Visualization/Vehicle XY Plotter/XY View ==
  Bus Element In2 : Inport  PortName=VehFdbk
  Bus Selector1 : BusSelector  OutputSignals=Body.InertFrm.Cg.Ang.phi,Body.InertFrm.Cg.Ang.theta,Body.InertFrm.Cg.Ang.psi  OutputAsBus=on
  Bus Selector10 : BusSelector  OutputSignals=Wheels.Wheels.Fx,Wheels.Wheels.Fy
  Bus Selector5 : BusSelector  OutputSignals=Steering.Front.WhlAng.FL,Steering.Front.WhlAng.FR,Steering.Rear.WhlAng.RL,Steering.Rear.WhlAng.RR  OutputAsBus=on
  Bus Selector6 : BusSelector  OutputSignals=Body.InertFrm.Geom.Disp.X,Body.InertFrm.Geom.Disp.Y,Body.InertFrm.Geom.Disp.Z  OutputAsBus=on
  Bus Selector7 : BusSelector  OutputSignals=Body.InertFrm.Geom.Vel.Xdot,Body.InertFrm.Geom.Vel.Ydot,Body.InertFrm.Geom.Vel.Zdot  OutputAsBus=on
  Bus Selector9 : BusSelector  OutputSignals=Driveline.EngSpd,Driveline.TransInfo.TransInfo.Trans.TransGear  OutputAsBus=on
  Bus to Vector{,1..4} (5 alike) : BusToVector
  Vehicle XY Plotter : vehdynlibviscommon/Vehicle XY Plot Configuration  extRef=off  extStats=on  extTireF=on  a=PlntVehDstCGFrntAxl  b=PlntVehDstCGRearAxl  w=PlntVehTrckWdth(1)  figBorder=10  bufferSize=1024  velNorm=5  tireFNorm=1000  pltDT=.1
  wires:
  Bus Selector7/1 -> Bus to Vector1/1
  Bus Selector5/1 -> Bus to Vector4/1
  Bus Selector10/2 -> Vehicle XY Plotter/7  "<Fy>"
  Bus to Vector1/1 -> Vehicle XY Plotter/3
  Bus Selector10/1 -> Vehicle XY Plotter/6  "<Fx>"
  Bus Selector1/1 -> Bus to Vector2/1
  Bus Selector9/1 -> Bus to Vector3/1
  Bus to Vector3/1 -> Vehicle XY Plotter/5
  Bus to Vector/1 -> Vehicle XY Plotter/1
  Bus Selector6/1 -> Bus to Vector/1
  Bus to Vector2/1 -> Vehicle XY Plotter/2
  Bus Element In2/1 -> Bus Selector10/1, Bus Selector9/1, Bus Selector5/1, Bus Selector7/1, Bus Selector1/1, Bus Selector6/1  "VehFdbk"
  Bus to Vector4/1 -> Vehicle XY Plotter/4

== system SparkEV/Visualization/Vehicle XY Plotter/XY View Ref ==
  Bus Element In2 : Inport  PortName=VehFdbk
  Bus Element In1 : Inport  Port=2  PortName=Ref  Element=YRef
  Bus Element In3 : Inport  Port=2  PortName=Ref  Element=XRef
  Bus Selector1 : BusSelector  OutputSignals=Body.InertFrm.Cg.Ang.phi,Body.InertFrm.Cg.Ang.theta,Body.InertFrm.Cg.Ang.psi  OutputAsBus=on
  Bus Selector10 : BusSelector  OutputSignals=Wheels.Wheels.Fx,Wheels.Wheels.Fy
  Bus Selector5 : BusSelector  OutputSignals=Steering.Front.WhlAng.FL,Steering.Front.WhlAng.FR,Steering.Rear.WhlAng.RL,Steering.Rear.WhlAng.RR  OutputAsBus=on
  Bus Selector6 : BusSelector  OutputSignals=Body.InertFrm.Geom.Disp.X,Body.InertFrm.Geom.Disp.Y,Body.InertFrm.Geom.Disp.Z  OutputAsBus=on
  Bus Selector7 : BusSelector  OutputSignals=Body.InertFrm.Geom.Vel.Xdot,Body.InertFrm.Geom.Vel.Ydot,Body.InertFrm.Geom.Vel.Zdot  OutputAsBus=on
  Bus Selector9 : BusSelector  OutputSignals=Driveline.EngSpd,Driveline.TransInfo.TransInfo.Trans.TransGear  OutputAsBus=on
  Bus to Vector{,1..3} (4 alike) : BusToVector
  Ground1 : Ground
  Mux : Mux  Inputs=3
  Vehicle XY Plotter : vehdynlibviscommon/Vehicle XY Plot Configuration  extRef=on  extStats=on  extTireF=on  a=PlntVehDstCGFrntAxl  b=PlntVehDstCGRearAxl  w=PlntVehTrckWdth(1)  figBorder=10  bufferSize=1024  velNorm=5  tireFNorm=1000  pltDT=.1
  wires:
  Bus Selector7/1 -> Bus to Vector1/1
  Bus Selector5/1 -> Vehicle XY Plotter/4
  Ground1/1 -> Mux/3
  Bus Selector10/2 -> Vehicle XY Plotter/8  "<Fy>"
  Bus to Vector1/1 -> Vehicle XY Plotter/3
  Bus Selector10/1 -> Vehicle XY Plotter/7  "<Fx>"
  Bus Selector1/1 -> Bus to Vector2/1
  Bus Selector9/1 -> Bus to Vector3/1
  Bus Element In1/1 -> Mux/2
  Bus to Vector3/1 -> Vehicle XY Plotter/6
  Bus Element In3/1 -> Mux/1
  Mux/1 -> Vehicle XY Plotter/5
  Bus to Vector/1 -> Vehicle XY Plotter/1
  Bus Selector6/1 -> Bus to Vector/1
  Bus to Vector2/1 -> Vehicle XY Plotter/2
  Bus Element In2/1 -> Bus Selector10/1, Bus Selector9/1, Bus Selector5/1, Bus Selector7/1, Bus Selector1/1, Bus Selector6/1  "VehFdbk"

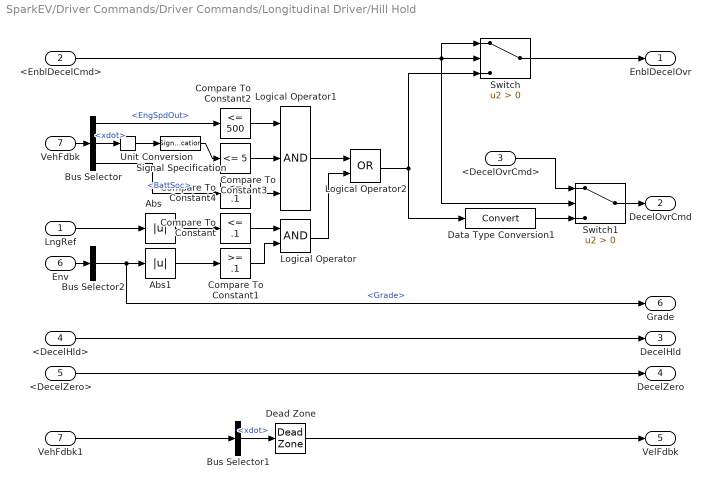
== system SparkEV/Driver Commands/Driver Commands/Longitudinal Driver/Hill Hold ==
  LngRef : Inport
  <EnblDecelCmd> : Inport  Port=2
  <DecelOvrCmd> : Inport  Port=3
  <DecelHld> : Inport  Port=4
  <DecelZero> : Inport  Port=5
  Env : Inport  Port=6
  VehFdbk : Inport  Port=7
  Abs : Abs  ZeroCross=off  SaturateOnIntegerOverflow=off
  Abs1 : Abs  ZeroCross=off  SaturateOnIntegerOverflow=off
  Bus Selector : BusSelector  OutputSignals=Engine.EngSpdOut,Body.BdyFrm.Cg.Vel.xdot,Battery.BattSoc
  Bus Selector1 : BusSelector  OutputSignals=Body.BdyFrm.Cg.Vel.xdot
  Bus Selector2 : BusSelector  OutputSignals=Grade
  Compare To Constant : simulink/Logic and Bit Operations/Compare To Constant  relop=<=  const=.1  OutDataTypeStr=boolean  ZeroCross=off
  Compare To Constant1 : simulink/Logic and Bit Operations/Compare To Constant  relop=>=  const=.1  OutDataTypeStr=boolean  ZeroCross=off
  Compare To Constant2 : simulink/Logic and Bit Operations/Compare To Constant  relop=<=  const=500  OutDataTypeStr=boolean  ZeroCross=off
  Compare To Constant3 : simulink/Logic and Bit Operations/Compare To Constant  relop=<=  const=5  OutDataTypeStr=boolean  ZeroCross=off
  Compare To Constant4 : simulink/Logic and Bit Operations/Compare To Constant  relop=<=  const=.1  OutDataTypeStr=boolean  ZeroCross=off
  Data Type Conversion1 : DataTypeConversion  SaturateOnIntegerOverflow=off  RndMeth=Floor
  Dead Zone : DeadZone  LowerValue=-.5  UpperValue=.5  ZeroCross=off
  Logical Operator : Logic  AllPortsSameDT=off  OutDataTypeStr=boolean
  Logical Operator1 : Logic  Inputs=3  AllPortsSameDT=off  OutDataTypeStr=boolean
  Logical Operator2 : Logic  Operator=OR  AllPortsSameDT=off  OutDataTypeStr=boolean
  Signal Specification : SignalSpecification  Unit=m/s
  Switch : Switch  Criteria=u2 > Threshold  SaturateOnIntegerOverflow=off  InputSameDT=off
  Switch1 : Switch  Criteria=u2 > Threshold  SaturateOnIntegerOverflow=off  InputSameDT=off
  Unit Conversion : UnitConversion
  VehFdbk1 : InportShadow  Port=7
  EnblDecelOvr : Outport
  DecelOvrCmd : Outport  Port=2
  DecelHld : Outport  Port=3
  DecelZero : Outport  Port=4
  VelFdbk : Outport  Port=5
  Grade : Outport  Port=6
  wires:
  Logical Operator2/1 -> Switch/3, Data Type Conversion1/1
  LngRef/1 -> Abs/1
  Abs/1 -> Compare To Constant/1
  Compare To Constant/1 -> Logical Operator/1
  Abs1/1 -> Compare To Constant1/1
  Compare To Constant1/1 -> Logical Operator/2
  Compare To Constant2/1 -> Logical Operator1/1
  Compare To Constant3/1 -> Logical Operator1/2
  Logical Operator1/1 -> Logical Operator2/1
  Logical Operator/1 -> Logical Operator2/2
  Compare To Constant4/1 -> Logical Operator1/3
  VehFdbk/1 -> Bus Selector/1
  Bus Selector/1 -> Compare To Constant2/1  "<EngSpdOut>"
  Bus Selector/2 -> Unit Conversion/1  "<xdot>"
  Bus Selector/3 -> Compare To Constant4/1  "<BattSoc>"
  Data Type Conversion1/1 -> Switch1/3
  <EnblDecelCmd>/1 -> Switch1/2, Switch/1, Switch/2
  Switch/1 -> EnblDecelOvr/1
  <DecelOvrCmd>/1 -> Switch1/1
  Switch1/1 -> DecelOvrCmd/1
  Env/1 -> Bus Selector2/1
  Bus Selector2/1 -> Grade/1, Abs1/1  "<Grade>"
  VehFdbk1/1 -> Bus Selector1/1
  Bus Selector1/1 -> Dead Zone/1  "<xdot>"
  Dead Zone/1 -> VelFdbk/1
  <DecelZero>/1 -> DecelZero/1
  <DecelHld>/1 -> DecelHld/1
  Unit Conversion/1 -> Signal Specification/1
  Signal Specification/1 -> Compare To Constant3/1

== system SparkEV/Driver Commands/Driver Commands/Predictive Driver/Hill Hold ==
  LngRef : Inport
  <EnblDecelCmd> : Inport  Port=2
  <DecelOvrCmd> : Inport  Port=3
  <DecelHld> : Inport  Port=4
  <DecelZero> : Inport  Port=5
  Env : Inport  Port=6
  VehFdbk : Inport  Port=7
  Abs : Abs  ZeroCross=off  SaturateOnIntegerOverflow=off
  Abs1 : Abs  ZeroCross=off  SaturateOnIntegerOverflow=off
  Bus Selector : BusSelector  OutputSignals=Engine.EngSpdOut,Body.BdyFrm.Cg.Vel.xdot,Battery.BattSoc
  Bus Selector1 : BusSelector  OutputSignals=Body.BdyFrm.Cg.Vel.xdot
  Bus Selector2 : BusSelector  OutputSignals=Grade
  Compare To Constant : simulink/Logic and Bit Operations/Compare To Constant  relop=<=  const=.1  OutDataTypeStr=boolean  ZeroCross=off
  Compare To Constant1 : simulink/Logic and Bit Operations/Compare To Constant  relop=>=  const=.1  OutDataTypeStr=boolean  ZeroCross=off
  Compare To Constant2 : simulink/Logic and Bit Operations/Compare To Constant  relop=<=  const=500  OutDataTypeStr=boolean  ZeroCross=off
  Compare To Constant3 : simulink/Logic and Bit Operations/Compare To Constant  relop=<=  const=5  OutDataTypeStr=boolean  ZeroCross=off
  Compare To Constant4 : simulink/Logic and Bit Operations/Compare To Constant  relop=<=  const=.1  OutDataTypeStr=boolean  ZeroCross=off
  Data Type Conversion1 : DataTypeConversion  SaturateOnIntegerOverflow=off  RndMeth=Floor
  Dead Zone : DeadZone  UpperValue=.5  ZeroCross=off
  Logical Operator : Logic  AllPortsSameDT=off  OutDataTypeStr=boolean
  Logical Operator1 : Logic  Inputs=3  AllPortsSameDT=off  OutDataTypeStr=boolean
  Logical Operator2 : Logic  Operator=OR  AllPortsSameDT=off  OutDataTypeStr=boolean
  Signal Specification : SignalSpecification  Unit=m/s
  Switch : Switch  Criteria=u2 > Threshold  SaturateOnIntegerOverflow=off  InputSameDT=off
  Switch1 : Switch  Criteria=u2 > Threshold  SaturateOnIntegerOverflow=off  InputSameDT=off
  Unit Conversion : UnitConversion
  VehFdbk1 : InportShadow  Port=7
  EnblDecelOvr : Outport
  DecelOvrCmd : Outport  Port=2
  DecelHld : Outport  Port=3
  DecelZero : Outport  Port=4
  Grade : Outport  Port=5
  VelFdbk : Outport  Port=6
  wires:
  Logical Operator2/1 -> Switch/3, Data Type Conversion1/1
  LngRef/1 -> Abs/1
  Abs/1 -> Compare To Constant/1
  Compare To Constant/1 -> Logical Operator/1
  Abs1/1 -> Compare To Constant1/1
  Compare To Constant1/1 -> Logical Operator/2
  Compare To Constant2/1 -> Logical Operator1/1
  Compare To Constant3/1 -> Logical Operator1/2
  Logical Operator1/1 -> Logical Operator2/1
  Logical Operator/1 -> Logical Operator2/2
  Compare To Constant4/1 -> Logical Operator1/3
  VehFdbk/1 -> Bus Selector/1
  Bus Selector/1 -> Compare To Constant2/1  "<EngSpdOut>"
  Bus Selector/3 -> Compare To Constant4/1  "<BattSoc>"
  Data Type Conversion1/1 -> Switch1/3
  <EnblDecelCmd>/1 -> Switch1/2, Switch/1, Switch/2
  Switch/1 -> EnblDecelOvr/1
  <DecelOvrCmd>/1 -> Switch1/1
  Switch1/1 -> DecelOvrCmd/1
  Env/1 -> Bus Selector2/1
  Bus Selector2/1 -> Grade/1, Abs1/1  "<Grade>"
  VehFdbk1/1 -> Bus Selector1/1
  Bus Selector1/1 -> Dead Zone/1  "<xdot>"
  Dead Zone/1 -> VelFdbk/1
  <DecelZero>/1 -> DecelZero/1
  <DecelHld>/1 -> DecelHld/1
  Unit Conversion/1 -> Signal Specification/1
  Bus Selector/2 -> Unit Conversion/1  "<xdot>"
  Signal Specification/1 -> Compare To Constant3/1

== system SparkEV/Environment/Ground Feedback/3D Engine/3D Engine Source ==
  WheelFdbk : Inport
  Multiple Points : Subsystem  VariantControl=terrType==2
  Single Point : Subsystem  VariantControl=terrType ==1
  z : Outport
  DCM : Outport  Port=2

== system SparkEV/Environment/Varying Friction/Varying Friction/Road Track Friction ==
  XWhl : Inport
  YWhl : Inport  Port=2
  Cg : Inport  Port=3
  2D Lookup Tbl for Scaling Fctr (Lambda) : Subsystem  TreatAsAtomicUnit=on
      mask init:
      | [~]=vehdynicon('vehdynblk',gcb);
  Bus Selector : BusSelector  OutputSignals=X,Y
  Cnst Lambda : Constant  Value=ones(4,1).*lambda_g
  Constant1 : Constant  Value=SplitLambdaTrck
  Creating Inertial Frm Bpt : Subsystem
  En at t = 0 : Subsystem
  "Lambda (t = 0) " : Memory  InitialCondition=ones(4,1).*lambda_g  InheritSampleTime=on
  Switch : Switch  Criteria=u2 > Threshold  SaturateOnIntegerOverflow=off  InputSameDT=off
  FricCoeffLambda : Outport
  wires:
  YWhl/1 -> 2D Lookup Tbl for Scaling Fctr (Lambda)/2(YWhl)
  XWhl/1 -> 2D Lookup Tbl for Scaling Fctr (Lambda)/1(XWhl)
  2D Lookup Tbl for Scaling Fctr (Lambda)/1(Lambda for each whl) -> Switch/1
  "Lambda (t = 0) "/1 -> FricCoeffLambda/1
  Switch/1 -> "Lambda (t = 0) "/1
  Cnst Lambda/1 -> Switch/3
  Constant1/1 -> Switch/2
  Cg/1 -> Bus Selector/1
  Creating Inertial Frm Bpt/1(XBpt) -> 2D Lookup Tbl for Scaling Fctr (Lambda)/3(XBpt)
  Creating Inertial Frm Bpt/2(YBpt) -> 2D Lookup Tbl for Scaling Fctr (Lambda)/4(YBpt)
  Bus Selector/1 -> Creating Inertial Frm Bpt/1(XCg)  "<X>"
  Bus Selector/2 -> Creating Inertial Frm Bpt/2(YCg)  "<Y>"
  En at t = 0/1(Out1) -> Creating Inertial Frm Bpt/Enable
